simulink model "integration_MPC_model_7"  (R2023a)
settings: Solver=VariableStepAuto  StartTime=0.0  StopTime=30  FixedStep=SampleTime  RelTol=1e-3
PreLoadFcn:
  | %
  | 
  | %   Copyright 2020-2022 The MathWorks, Inc.
  | 
  | %Based on the quadcopter model used in jMAVSim
  | 
  | Ixx = 0.005; %Kgm^2
  | Iyy = 0.005;
  | Izz = 0.009;
  | 
  | 
  | inertia = diag([Ixx, Iyy, Izz]);
  | 
  | mass = 0.8; %Kg
  | g = 9.81; %m/s^2
  | 
  | armLength = 0.33/2; % length of Arm measured from center in m
  | 
  | rotorThrustMax = 4; %N
  | 
  | rotorTorqueMax = 0.05 ;%Nm
  | 
  | rotorTimeConst = 0.005 ;% time constant of rotor (motor + propeller)
  | 
  | %rotorOffset = [0 0 0]; % Rotors position offsets from Gravity center
  | 
  | dragCoeffMov = 0.01; %drag coefficient for linear motion of quadcopter
  | windVel = [0 0 0]';
  | 
  | % Initial states
  | init.posNED = [0, 0, 0]; % m
  | init.vb = [0 0 0]'; %m/s
  | init.euler = [0, 0, 0]'; %Roll Pitch Yaw Rads
  | init.angRates = [0, 0, 0]; %rad/s
  | 
  | 
  | %Computed from above values
  | rotorPositions = zeros(3,4);
  | axisD = armLength/sqrt(2);
  | rotorPositions(:,1) = [axisD, axisD, 0]';
  | rotorPositions(:,2) = [-axisD, -axisD, 0]';
  | rotorPositions(:,3) = [+axisD, -axisD, 0]';
  | rotorPositions(:,4) = [-axisD, axisD, 0]';
  | rotorDir = [-1, -1, 1, 1]; %rotation direction. +ve = clockwise
  | 
  | % Sample Time
  | SampleTime = 0.008;
  | 
  | %Gain to convert m to mm
  | m_to_mm = 1000;
  | 
  | %Gain to convert m/s^2 to mG
  | ms2_to_mg = (1/9.80665)*1000;
  | 
  | %Gain to convert m/s to cm/s
  | ms_to_cms = 100;
  | 
  | %Reference height for 'Flat Earth to LLA'
  | ref_height = -71.3232;
  | 
  | ... (+137 lines)
values from neighbouring files (symbols this model uses):
  a = 6    [integration_parameters.m]    (also in simulation_parameters.m)
  delay_tilt = 0.004    [integration_parameters.m]    (also in simulation_parameters.m)
  J = diag([0.018 0.035 0.051])    [integration_parameters.m]    (also in simulation_parameters.m)
  kf = 65    [integration_parameters.m]    (also in simulation_parameters.m)
  Lh = 0.2    [CoG_shift.m]    (also in integration_parameters.m; simulation_parameters.m)
  Lv = 0.2    [integration_parameters.m]    (also in simulation_parameters.m)
  m = 1.12    [integration_parameters.m]    (also in optimal_controller_pitching.m; simulation_parameters.m)
  N = 150    [MPC_controller_full.m]
  p_D = 0    [controller_parameters.m]    (also in integration_parameters.m)
  p_I = 0    [controller_parameters.m]    (also in integration_parameters.m)
  p_P = 0.35    [controller_parameters.m]    (also in integration_parameters.m)
  pitch_D = 0    [controller_parameters.m]    (also in integration_parameters.m)
  pitch_I = 0.05    [controller_parameters.m]    (also in integration_parameters.m = 0)
  pitch_P = 2    [controller_parameters.m]    (also in integration_parameters.m = 10)
  reference = [1 1 1 0 30 60]'    [integration_parameters.m]    (also in simulation_parameters.m = [1 1 1 0 30 40]')
  roll_D = 1    [controller_parameters.m]    (also in integration_parameters.m)
  roll_I = 0    [controller_parameters.m]    (also in integration_parameters.m)
  roll_P = 8    [controller_parameters.m]    (also in integration_parameters.m)
  s_r = [1 1 1 1 1 1]    [integration_parameters.m]    (also in simulation_parameters.m)
  Tmax = 5.5    [integration_parameters.m]    (also in simulation_parameters.m)
  toll = 1e-12    [integration_parameters.m]    (also in simulation_parameters.m)
  vy_D = 0    [controller_parameters.m]    (also in integration_parameters.m)
  vy_I = 0    [controller_parameters.m]    (also in integration_parameters.m)
  vy_P = 12    [controller_parameters.m]    (also in integration_parameters.m)
  vz_D = 0    [controller_parameters.m]    (also in integration_parameters.m)
  vz_I = 0    [controller_parameters.m]    (also in integration_parameters.m)
  vz_P = 8    [controller_parameters.m]    (also in integration_parameters.m = 9)
  x_D = 1.5    [controller_parameters.m]    (also in integration_parameters.m = 0)
  x_I = 0    [controller_parameters.m]    (also in integration_parameters.m)
  x_P = 6    [controller_parameters.m]    (also in integration_parameters.m = 1.5)
  y_D = 0.3    [controller_parameters.m]    (also in integration_parameters.m)
  y_I = 0    [controller_parameters.m]    (also in integration_parameters.m)
  y_P = 1.5    [controller_parameters.m]    (also in integration_parameters.m)
  yaw_D = 0    [controller_parameters.m]    (also in integration_parameters.m)
  yaw_I = 0    [controller_parameters.m]    (also in integration_parameters.m)
  yaw_P = 1.5    [controller_parameters.m]    (also in integration_parameters.m)
  z_D = 0    [controller_parameters.m]    (also in integration_parameters.m)
  z_I = 0    [controller_parameters.m]    (also in integration_parameters.m)
  z_P = 3    [controller_parameters.m]    (also in integration_parameters.m = 2.5)
undefined symbols (not defined in the file or in its folder): X, Y, Z
libraries: sm_lib x49, nesl_utility x29, slpidlib x9, simulink x5, simulink_extras x3, SignalEditorBlockLib x1, mpclib x1, eeGeneralControl x1
(part 3 of 4)

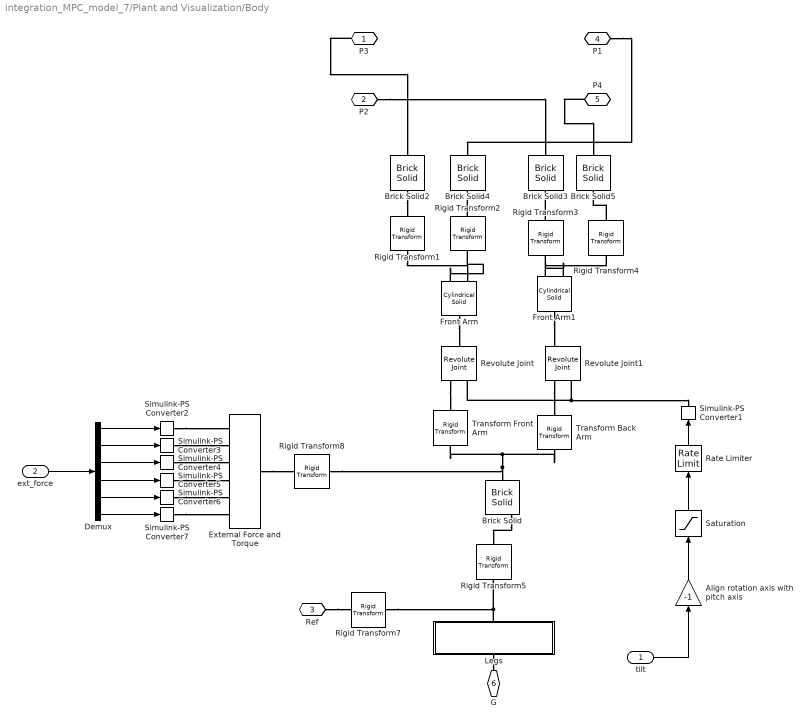
== system integration_MPC_model_7/Plant and Visualization/Body ==
  tilt : Inport
  ext_force : Inport  Port=2
  Align rotation axis with pitch axis : Gain  Gain=-1
  Brick Solid : sm_lib/Body Elements/Brick Solid  GraphicAmbientColor=[0.15 0.15 0.15 1.0]  BasedOnType=Mass  BrickDimensions=[0.1 0.5 0.05]  BrickDimensionsUnits=m  CenterOfMass=[0 0 0]  CenterOfMassUnits=m  GraphicDiffuseColor=[0.5 0.5 0.5]  Density=50  DensityUnits=kg/m^3  DoExposeReferenceFrame=on  GraphicEmissiveColor=[0.0 0.0 0.0 1.0]  ExportEntireGeometry=off  SerializedFrames=<Frames><Frame><Id>Frame2</Id><Value><Name>top</Name><Origin><Source>GeometricFeature</Source><FeatureName>+z surface</FeatureName></Origin><PrimaryAxis><DefinedDirection>+Z</DefinedDirection><Source>ReferenceFrame</Source><SourceDirection>+Z</SourceDirection><FeatureName></FeatureName></PrimaryAxis><SecondaryAxis><DefinedDirection>+X</DefinedDirection><Source>ReferenceFrame</Source><SourceDirection>+Y</SourceDirection><FeatureName></FeatureName></SecondaryAxis></Value></Frame><Frame><Id>Frame3</Id><Value><Name>bottom</Name><Origin><Source>GeometricFeature</Source><FeatureName>-z surface</FeatureName></Origin><PrimaryAxis><DefinedDirection>+Z</DefinedDirection><Source>ReferenceFrame</Source><SourceDirection>+Z</SourceDirection><FeatureName></FeatureName></PrimaryAxis><SecondaryAxis><DefinedDirection>+X</DefinedDirection><Source>ReferenceFrame</Source><SourceDirection>+X</SourceDirection><FeatureName></FeatureName></SecondaryAxis></Value></Frame></Frames>  MarkerShape=Sphere  MarkerSize=10  GraphicType=FromGeometry  InertiaType=CalculateFromGeometry  Mass=0.5  MassUnits=kg  MomentsOfInertia=[1 1 1]  MomentsOfInertiaUnits=kg*m^2  GraphicOpacity=1.0  ProductsOfInertia=[0 0 0]  ProductsOfInertiaUnits=kg*m^2  GraphicShininess=75  GraphicSpecularColor=[0.5 0.5 0.5 1.0]  GraphicVisPropType=AdvancedVisualProperties
  Brick Solid2 : sm_lib/Body Elements/Brick Solid  GraphicAmbientColor=[0.15 0.15 0.15 1.0]  BasedOnType=Mass  BrickDimensions=[0.04 0.04 0.04]  BrickDimensionsUnits=m  CenterOfMass=[0 0 0]  CenterOfMassUnits=m  GraphicDiffuseColor=[1.0 0.6 0.6]  Density=0.00001  DensityUnits=kg/m^3  DoExposeReferenceFrame=on  GraphicEmissiveColor=[0.0 0.0 0.0 1.0]  ExportEntireGeometry=off  SerializedFrames=<Frames><Frame><Id>Frame1</Id><Value><Name>top</Name><Origin><Source>GeometricFeature</Source><FeatureName>+z surface</FeatureName></Origin><PrimaryAxis><DefinedDirection>+Z</DefinedDirection><Source>ReferenceFrame</Source><SourceDirection>+Z</SourceDirection><FeatureName></FeatureName></PrimaryAxis><SecondaryAxis><DefinedDirection>+X</DefinedDirection><Source>ReferenceFrame</Source><SourceDirection>+X</SourceDirection><FeatureName></FeatureName></SecondaryAxis></Value></Frame></Frames>  MarkerShape=Sphere  MarkerSize=10  GraphicType=FromGeometry  InertiaType=CalculateFromGeometry  Mass=0.08  MassUnits=kg  MomentsOfInertia=[1 1 1]  MomentsOfInertiaUnits=kg*m^2  GraphicOpacity=1.0  ProductsOfInertia=[0 0 0]  ProductsOfInertiaUnits=kg*m^2  GraphicShininess=75  GraphicSpecularColor=[0.5 0.5 0.5 1.0]  GraphicVisPropType=SimpleVisualProperties
  Brick Solid3 : sm_lib/Body Elements/Brick Solid  GraphicAmbientColor=[0.15 0.15 0.15 1.0]  BasedOnType=Mass  BrickDimensions=[0.04 0.04 0.04]  BrickDimensionsUnits=m  CenterOfMass=[0 0 0]  CenterOfMassUnits=m  GraphicDiffuseColor=[0.4 1.0 0.4]  Density=0.00001  DensityUnits=kg/m^3  DoExposeReferenceFrame=on  GraphicEmissiveColor=[0.0 0.0 0.0 1.0]  ExportEntireGeometry=off  SerializedFrames=<Frames><Frame><Id>Frame1</Id><Value><Name>top</Name><Origin><Source>GeometricFeature</Source><FeatureName>+z surface</FeatureName></Origin><PrimaryAxis><DefinedDirection>+Z</DefinedDirection><Source>ReferenceFrame</Source><SourceDirection>+Z</SourceDirection><FeatureName></FeatureName></PrimaryAxis><SecondaryAxis><DefinedDirection>+X</DefinedDirection><Source>ReferenceFrame</Source><SourceDirection>+X</SourceDirection><FeatureName></FeatureName></SecondaryAxis></Value></Frame></Frames>  MarkerShape=Sphere  MarkerSize=10  GraphicType=FromGeometry  InertiaType=CalculateFromGeometry  Mass=0.08  MassUnits=kg  MomentsOfInertia=[1 1 1]  MomentsOfInertiaUnits=kg*m^2  GraphicOpacity=1.0  ProductsOfInertia=[0 0 0]  ProductsOfInertiaUnits=kg*m^2  GraphicShininess=75  GraphicSpecularColor=[0.5 0.5 0.5 1.0]  GraphicVisPropType=SimpleVisualProperties
  Brick Solid4 : sm_lib/Body Elements/Brick Solid  GraphicAmbientColor=[0.15 0.15 0.15 1.0]  BasedOnType=Mass  BrickDimensions=[0.04 0.04 0.04]  BrickDimensionsUnits=m  CenterOfMass=[0 0 0]  CenterOfMassUnits=m  GraphicDiffuseColor=[0.0 0.6 1.0]  Density=0.00001  DensityUnits=kg/m^3  DoExposeReferenceFrame=on  GraphicEmissiveColor=[0.0 0.0 0.0 1.0]  ExportEntireGeometry=off  SerializedFrames=<Frames><Frame><Id>Frame1</Id><Value><Name>top</Name><Origin><Source>GeometricFeature</Source><FeatureName>+z surface</FeatureName></Origin><PrimaryAxis><DefinedDirection>+Z</DefinedDirection><Source>ReferenceFrame</Source><SourceDirection>+Z</SourceDirection><FeatureName></FeatureName></PrimaryAxis><SecondaryAxis><DefinedDirection>+X</DefinedDirection><Source>ReferenceFrame</Source><SourceDirection>+X</SourceDirection><FeatureName></FeatureName></SecondaryAxis></Value></Frame></Frames>  MarkerShape=Sphere  MarkerSize=10  GraphicType=FromGeometry  InertiaType=CalculateFromGeometry  Mass=0.08  MassUnits=kg  MomentsOfInertia=[1 1 1]  MomentsOfInertiaUnits=kg*m^2  GraphicOpacity=1.0  ProductsOfInertia=[0 0 0]  ProductsOfInertiaUnits=kg*m^2  GraphicShininess=75  GraphicSpecularColor=[0.5 0.5 0.5 1.0]  GraphicVisPropType=SimpleVisualProperties
  Brick Solid5 : sm_lib/Body Elements/Brick Solid  GraphicAmbientColor=[0.15 0.15 0.15 1.0]  BasedOnType=Mass  BrickDimensions=[0.04 0.04 0.04]  BrickDimensionsUnits=m  CenterOfMass=[0 0 0]  CenterOfMassUnits=m  GraphicDiffuseColor=[0.5 0.5 0.5]  Density=0.00001  DensityUnits=kg/m^3  DoExposeReferenceFrame=on  GraphicEmissiveColor=[0.0 0.0 0.0 1.0]  ExportEntireGeometry=off  SerializedFrames=<Frames><Frame><Id>Frame1</Id><Value><Name>top</Name><Origin><Source>GeometricFeature</Source><FeatureName>+z surface</FeatureName></Origin><PrimaryAxis><DefinedDirection>+Z</DefinedDirection><Source>ReferenceFrame</Source><SourceDirection>+Z</SourceDirection><FeatureName></FeatureName></PrimaryAxis><SecondaryAxis><DefinedDirection>+X</DefinedDirection><Source>ReferenceFrame</Source><SourceDirection>+X</SourceDirection><FeatureName></FeatureName></SecondaryAxis></Value></Frame></Frames>  MarkerShape=Sphere  MarkerSize=10  GraphicType=FromGeometry  InertiaType=CalculateFromGeometry  Mass=0.08  MassUnits=kg  MomentsOfInertia=[1 1 1]  MomentsOfInertiaUnits=kg*m^2  GraphicOpacity=1.0  ProductsOfInertia=[0 0 0]  ProductsOfInertiaUnits=kg*m^2  GraphicShininess=75  GraphicSpecularColor=[0.5 0.5 0.5 1.0]  GraphicVisPropType=SimpleVisualProperties
  Demux : Demux  Outputs=6
  External Force and Torque : sm_lib/Forces and Torques/External Force and Torque  ForceResolutionFrame=AttachedFrame  EnableForceX=on  EnableForceY=on  EnableForceZ=on  EnableForce=off  TorqueResolutionFrame=AttachedFrame  EnableTorqueX=on  EnableTorqueY=on  EnableTorqueZ=on  EnableTorque=off
  Front Arm : sm_lib/Body Elements/Cylindrical Solid  GraphicAmbientColor=[0.15 0.15 0.15 1.0]  BasedOnType=Mass  CenterOfMass=[0 0 0]  CenterOfMassUnits=m  GraphicDiffuseColor=[1.0 0.0 0.2]  CylinderLength=0.4  CylinderLengthUnits=m  CylinderRadius=0.016  CylinderRadiusUnits=m  Density=0.0003  DensityUnits=g/cm^3  DoExposeReferenceFrame=on  GraphicEmissiveColor=[0.0 0.0 0.0 1.0]  ExportEntireGeometry=off  SerializedFrames=<Frames><Frame><Id>Frame1</Id><Value><Name>right</Name><Origin><Source>GeometricFeature</Source><FeatureName>top curve</FeatureName></Origin><PrimaryAxis><DefinedDirection>+Z</DefinedDirection><Source>ReferenceFrame</Source><SourceDirection>+Z</SourceDirection><FeatureName></FeatureName></PrimaryAxis><SecondaryAxis><DefinedDirection>+X</DefinedDirection><Source>ReferenceFrame</Source><SourceDirection>+X</SourceDirection><FeatureName></FeatureName></SecondaryAxis></Value></Frame><Frame><Id>Frame2</Id><Value><Name>left</Name><Origin><Source>GeometricFeature</Source><FeatureName>bottom curve</FeatureName></Origin><PrimaryAxis><DefinedDirection>+Z</DefinedDirection><Source>ReferenceFrame</Source><SourceDirection>+Z</SourceDirection><FeatureName></FeatureName></PrimaryAxis><SecondaryAxis><DefinedDirection>+X</DefinedDirection><Source>ReferenceFrame</Source><SourceDirection>+X</SourceDirection><FeatureName></FeatureName></SecondaryAxis></Value></Frame></Frames>  MarkerShape=Sphere  MarkerSize=10  GraphicType=FromGeometry  InertiaType=CalculateFromGeometry  Mass=0.1  MassUnits=kg  MomentsOfInertia=[1 1 1]  MomentsOfInertiaUnits=kg*m^2  GraphicOpacity=1.0  ProductsOfInertia=[0 0 0]  ProductsOfInertiaUnits=kg*m^2  GraphicShininess=75  GraphicSpecularColor=[0.5 0.5 0.5 1.0]  GraphicVisPropType=SimpleVisualProperties
  Front Arm1 : sm_lib/Body Elements/Cylindrical Solid  GraphicAmbientColor=[0.15 0.15 0.15 1.0]  BasedOnType=Mass  CenterOfMass=[0 0 0]  CenterOfMassUnits=m  GraphicDiffuseColor=[1.0 0.0 0.2]  CylinderLength=0.4  CylinderLengthUnits=m  CylinderRadius=0.016  CylinderRadiusUnits=m  Density=0.0003  DensityUnits=g/cm^3  DoExposeReferenceFrame=on  GraphicEmissiveColor=[0.0 0.0 0.0 1.0]  ExportEntireGeometry=off  SerializedFrames=<Frames><Frame><Id>Frame1</Id><Value><Name>right</Name><Origin><Source>GeometricFeature</Source><FeatureName>top curve</FeatureName></Origin><PrimaryAxis><DefinedDirection>+Z</DefinedDirection><Source>ReferenceFrame</Source><SourceDirection>+Z</SourceDirection><FeatureName></FeatureName></PrimaryAxis><SecondaryAxis><DefinedDirection>+X</DefinedDirection><Source>ReferenceFrame</Source><SourceDirection>+X</SourceDirection><FeatureName></FeatureName></SecondaryAxis></Value></Frame><Frame><Id>Frame2</Id><Value><Name>left</Name><Origin><Source>GeometricFeature</Source><FeatureName>bottom curve</FeatureName></Origin><PrimaryAxis><DefinedDirection>+Z</DefinedDirection><Source>ReferenceFrame</Source><SourceDirection>+Z</SourceDirection><FeatureName></FeatureName></PrimaryAxis><SecondaryAxis><DefinedDirection>+X</DefinedDirection><Source>ReferenceFrame</Source><SourceDirection>+X</SourceDirection><FeatureName></FeatureName></SecondaryAxis></Value></Frame></Frames>  MarkerShape=Sphere  MarkerSize=10  GraphicType=FromGeometry  InertiaType=CalculateFromGeometry  Mass=0.1  MassUnits=kg  MomentsOfInertia=[1 1 1]  MomentsOfInertiaUnits=kg*m^2  GraphicOpacity=1.0  ProductsOfInertia=[0 0 0]  ProductsOfInertiaUnits=kg*m^2  GraphicShininess=75  GraphicSpecularColor=[0.5 0.5 0.5 1.0]  GraphicVisPropType=SimpleVisualProperties
  Legs : Subsystem
  Rate Limiter : RateLimiter  RisingSlewLimit=4.2  FallingSlewLimit=-4.2
  Revolute Joint : sm_lib/Joints/Revolute Joint  JointMode=Normal  SenseConstraintForce=off  SenseConstraintForceX=off  SenseConstraintForceY=off  SenseConstraintForceZ=off  SenseConstraintTorque=off  SenseConstraintTorqueX=off  SenseConstraintTorqueY=off  SenseConstraintTorqueZ=off  SenseTotalForce=off  SenseTotalForceX=off  SenseTotalForceY=off  SenseTotalForceZ=off  SenseTotalTorque=off  SenseTotalTorqueX=off  SenseTotalTorqueY=off  SenseTotalTorqueZ=off  CompositeWrenchDir=FollowerOnBase  CompositeWrenchFrame=BaseFrame  EquilibriumPosition=0  EquilibriumPositionUnits=deg  SpringStiffness=0  SpringStiffnessUnits=N*m/deg  DampingCoefficient=0  DampingCoefficientUnits=N*m/(deg/s)  TorqueActuationMode=ComputedTorque  MotionActuationMode=InputMotion  SensePosition=off  SenseVelocity=off  SenseAcceleration=off  SenseTorqueForce=off  SenseLowerLimitTorqueForce=off  SenseUpperLimitTorqueForce=off  LowerLimitSpecify=on  LowerLimitBound=-45  LowerLimitBoundUnits=deg  LowerLimitStiffness=1e4  LowerLimitStiffnessUnits=N*m/deg  LowerLimitDamping=10  LowerLimitDampingUnits=N*m/(deg/s)  LowerLimitTransitionRegionWidth=0.1  LowerLimitTransitionRegionWidthUnits=deg  UpperLimitSpecify=on  UpperLimitBound=45  UpperLimitBoundUnits=deg  UpperLimitStiffness=1e4  UpperLimitStiffnessUnits=N*m/deg  UpperLimitDamping=10  UpperLimitDampingUnits=N*m/(deg/s)  UpperLimitTransitionRegionWidth=0.1  UpperLimitTransitionRegionWidthUnits=deg  PositionTargetSpecify=off  PositionTargetPriority=High  PositionTargetValue=0  PositionTargetValueUnits=deg  VelocityTargetSpecify=off  VelocityTargetPriority=High  VelocityTargetValue=0  VelocityTargetValueUnits=deg/s
  Revolute Joint1 : sm_lib/Joints/Revolute Joint  JointMode=Normal  SenseConstraintForce=off  SenseConstraintForceX=off  SenseConstraintForceY=off  SenseConstraintForceZ=off  SenseConstraintTorque=off  SenseConstraintTorqueX=off  SenseConstraintTorqueY=off  SenseConstraintTorqueZ=off  SenseTotalForce=off  SenseTotalForceX=off  SenseTotalForceY=off  SenseTotalForceZ=off  SenseTotalTorque=off  SenseTotalTorqueX=off  SenseTotalTorqueY=off  SenseTotalTorqueZ=off  CompositeWrenchDir=FollowerOnBase  CompositeWrenchFrame=BaseFrame  EquilibriumPosition=0  EquilibriumPositionUnits=deg  SpringStiffness=0  SpringStiffnessUnits=N*m/deg  DampingCoefficient=0  DampingCoefficientUnits=N*m/(deg/s)  TorqueActuationMode=ComputedTorque  MotionActuationMode=InputMotion  SensePosition=on  SenseVelocity=off  SenseAcceleration=off  SenseTorqueForce=off  SenseLowerLimitTorqueForce=off  SenseUpperLimitTorqueForce=off  LowerLimitSpecify=on  LowerLimitBound=-45  LowerLimitBoundUnits=deg  LowerLimitStiffness=1e4  LowerLimitStiffnessUnits=N*m/deg  LowerLimitDamping=10  LowerLimitDampingUnits=N*m/(deg/s)  LowerLimitTransitionRegionWidth=0.1  LowerLimitTransitionRegionWidthUnits=deg  UpperLimitSpecify=on  UpperLimitBound=45  UpperLimitBoundUnits=deg  UpperLimitStiffness=1e4  UpperLimitStiffnessUnits=N*m/deg  UpperLimitDamping=10  UpperLimitDampingUnits=N*m/(deg/s)  UpperLimitTransitionRegionWidth=0.1  UpperLimitTransitionRegionWidthUnits=deg  PositionTargetSpecify=off  PositionTargetPriority=High  PositionTargetValue=0  PositionTargetValueUnits=deg  VelocityTargetSpecify=off  VelocityTargetPriority=High  VelocityTargetValue=0  VelocityTargetValueUnits=deg/s
  Rigid Transform1 : sm_lib/Frames and Transforms/Rigid Transform  TranslationMethod=None  TranslationStandardOffset=0  TranslationStandardOffsetUnits=m  TranslationStandardAxis=+Z  TranslationCartesianOffset=[0.2 0 0]  TranslationCartesianOffsetUnits=m  TranslationROffset=0  TranslationROffsetUnits=m  TranslationZOffset=0  TranslationZOffsetUnits=m  TranslationThetaOffset=0  TranslationThetaOffsetUnits=deg  RotationMethod=RotationSequence  RotationAngleUnits=deg  RotationStandardAxis=+X  RotationAngle=180  RotationArbitraryAxis=[0 0 1]  FollAlignAxisA=+X  BaseAlignAxisA=+Y  FollAlignAxisB=+Y  BaseAlignAxisB=+Z  RotationSequenceAxes=FollowerAxes  RotationSequence=ZYZ  RotationSequenceAngles=[90 180 0]  RotationSequenceAnglesUnits=deg  RotationMatrix=[1 0 0; 0 1 0; 0 0 1]  Quaternion=[1 0 0 0]
  Rigid Transform2 : sm_lib/Frames and Transforms/Rigid Transform  TranslationMethod=None  TranslationStandardOffset=0  TranslationStandardOffsetUnits=m  TranslationStandardAxis=+Z  TranslationCartesianOffset=[0.2 0 0]  TranslationCartesianOffsetUnits=m  TranslationROffset=0  TranslationROffsetUnits=m  TranslationZOffset=0  TranslationZOffsetUnits=m  TranslationThetaOffset=0  TranslationThetaOffsetUnits=deg  RotationMethod=StandardAxis  RotationAngleUnits=deg  RotationStandardAxis=+Z  RotationAngle=90  RotationArbitraryAxis=[0 0 1]  FollAlignAxisA=+X  BaseAlignAxisA=+Y  FollAlignAxisB=+Y  BaseAlignAxisB=+Z  RotationSequenceAxes=FollowerAxes  RotationSequence=XYX  RotationSequenceAngles=[0 0 0]  RotationSequenceAnglesUnits=deg  RotationMatrix=[1 0 0; 0 1 0; 0 0 1]  Quaternion=[1 0 0 0]
  Rigid Transform3 : sm_lib/Frames and Transforms/Rigid Transform  TranslationMethod=None  TranslationStandardOffset=0  TranslationStandardOffsetUnits=m  TranslationStandardAxis=+Z  TranslationCartesianOffset=[0.2 0 0]  TranslationCartesianOffsetUnits=m  TranslationROffset=0  TranslationROffsetUnits=m  TranslationZOffset=0  TranslationZOffsetUnits=m  TranslationThetaOffset=0  TranslationThetaOffsetUnits=deg  RotationMethod=RotationSequence  RotationAngleUnits=deg  RotationStandardAxis=+X  RotationAngle=180  RotationArbitraryAxis=[0 0 1]  FollAlignAxisA=+X  BaseAlignAxisA=+Y  FollAlignAxisB=+Y  BaseAlignAxisB=+Z  RotationSequenceAxes=FollowerAxes  RotationSequence=ZYZ  RotationSequenceAngles=[90 180 0]  RotationSequenceAnglesUnits=deg  RotationMatrix=[1 0 0; 0 1 0; 0 0 1]  Quaternion=[1 0 0 0]
  Rigid Transform4 : sm_lib/Frames and Transforms/Rigid Transform  TranslationMethod=None  TranslationStandardOffset=0  TranslationStandardOffsetUnits=m  TranslationStandardAxis=+Z  TranslationCartesianOffset=[0.2 0 0]  TranslationCartesianOffsetUnits=m  TranslationROffset=0  TranslationROffsetUnits=m  TranslationZOffset=0  TranslationZOffsetUnits=m  TranslationThetaOffset=0  TranslationThetaOffsetUnits=deg  RotationMethod=StandardAxis  RotationAngleUnits=deg  RotationStandardAxis=+Z  RotationAngle=90  RotationArbitraryAxis=[0 0 1]  FollAlignAxisA=+X  BaseAlignAxisA=+Y  FollAlignAxisB=+Y  BaseAlignAxisB=+Z  RotationSequenceAxes=FollowerAxes  RotationSequence=XYX  RotationSequenceAngles=[0 0 0]  RotationSequenceAnglesUnits=deg  RotationMatrix=[1 0 0; 0 1 0; 0 0 1]  Quaternion=[1 0 0 0]
  Rigid Transform5 : sm_lib/Frames and Transforms/Rigid Transform  TranslationMethod=None  TranslationStandardOffset=0  TranslationStandardOffsetUnits=m  TranslationStandardAxis=+Z  TranslationCartesianOffset=[0 0 0]  TranslationCartesianOffsetUnits=m  TranslationROffset=0  TranslationROffsetUnits=m  TranslationZOffset=0  TranslationZOffsetUnits=m  TranslationThetaOffset=0  TranslationThetaOffsetUnits=deg  RotationMethod=RotationSequence  RotationAngleUnits=deg  RotationStandardAxis=-Z  RotationAngle=90  RotationArbitraryAxis=[0 0 1]  FollAlignAxisA=+X  BaseAlignAxisA=+Y  FollAlignAxisB=+Y  BaseAlignAxisB=+Z  RotationSequenceAxes=FollowerAxes  RotationSequence=ZYX  RotationSequenceAngles=[-90 180 0]  RotationSequenceAnglesUnits=deg  RotationMatrix=[1 0 0; 0 1 0; 0 0 1]  Quaternion=[1 0 0 0]
  Rigid Transform7 : sm_lib/Frames and Transforms/Rigid Transform  TranslationMethod=None  TranslationStandardOffset=0  TranslationStandardOffsetUnits=m  TranslationStandardAxis=+Z  TranslationCartesianOffset=[0 0 0]  TranslationCartesianOffsetUnits=m  TranslationROffset=0  TranslationROffsetUnits=m  TranslationZOffset=0  TranslationZOffsetUnits=m  TranslationThetaOffset=0  TranslationThetaOffsetUnits=deg  RotationMethod=StandardAxis  RotationAngleUnits=deg  RotationStandardAxis=+X  RotationAngle=180  RotationArbitraryAxis=[0 0 1]  FollAlignAxisA=+X  BaseAlignAxisA=+Y  FollAlignAxisB=+Y  BaseAlignAxisB=+Z  RotationSequenceAxes=FollowerAxes  RotationSequence=XYX  RotationSequenceAngles=[0 0 0]  RotationSequenceAnglesUnits=deg  RotationMatrix=[1 0 0; 0 1 0; 0 0 1]  Quaternion=[1 0 0 0]
  Rigid Transform8 : sm_lib/Frames and Transforms/Rigid Transform  TranslationMethod=None  TranslationStandardOffset=0  TranslationStandardOffsetUnits=m  TranslationStandardAxis=+Z  TranslationCartesianOffset=[0 0 0]  TranslationCartesianOffsetUnits=m  TranslationROffset=0  TranslationROffsetUnits=m  TranslationZOffset=0  TranslationZOffsetUnits=m  TranslationThetaOffset=0  TranslationThetaOffsetUnits=deg  RotationMethod=StandardAxis  RotationAngleUnits=deg  RotationStandardAxis=+Z  RotationAngle=90  RotationArbitraryAxis=[0 0 1]  FollAlignAxisA=+X  BaseAlignAxisA=+Y  FollAlignAxisB=+Y  BaseAlignAxisB=+Z  RotationSequenceAxes=FollowerAxes  RotationSequence=XYX  RotationSequenceAngles=[0 0 0]  RotationSequenceAnglesUnits=deg  RotationMatrix=[1 0 0; 0 1 0; 0 0 1]  Quaternion=[1 0 0 0]
  Saturation : Saturate  UpperLimit=1.6  LowerLimit=-1.6
  Simulink-PS Converter{1..7} (7 alike) : nesl_utility/Simulink-PS Converter  PhysicalDomain=network_engine_domain  SubClassName=ps_input  LeftPortType=input  RightPortType=output  PseudoPeriodic=off  Frequencies=[]  NoiseDistribution=none  NoiseParameters=[]  Unit=1  AffineConversion=off  FilteringAndDerivatives=filter  SimscapeFilterOrder=2  InputFilterTimeConstant=0.001  UdotUserProvided=0
  Transform Back Arm : sm_lib/Frames and Transforms/Rigid Transform  TranslationMethod=Cartesian  TranslationStandardOffset=0  TranslationStandardOffsetUnits=m  TranslationStandardAxis=+Z  TranslationCartesianOffset=[0 -0.2 0]  TranslationCartesianOffsetUnits=m  TranslationROffset=0  TranslationROffsetUnits=m  TranslationZOffset=0  TranslationZOffsetUnits=m  TranslationThetaOffset=0  TranslationThetaOffsetUnits=deg  RotationMethod=StandardAxis  RotationAngleUnits=deg  RotationStandardAxis=+Y  RotationAngle=90  RotationArbitraryAxis=[0 0 1]  FollAlignAxisA=+X  BaseAlignAxisA=+Y  FollAlignAxisB=+Y  BaseAlignAxisB=+Z  RotationSequenceAxes=FollowerAxes  RotationSequence=XYX  RotationSequenceAngles=[90 180 0]  RotationSequenceAnglesUnits=deg  RotationMatrix=[1 0 0; 0 1 0; 0 0 1]  Quaternion=[1 0 0 0]
  Transform Front Arm : sm_lib/Frames and Transforms/Rigid Transform  TranslationMethod=Cartesian  TranslationStandardOffset=0  TranslationStandardOffsetUnits=m  TranslationStandardAxis=+Z  TranslationCartesianOffset=[0 0.2 0]  TranslationCartesianOffsetUnits=m  TranslationROffset=0  TranslationROffsetUnits=m  TranslationZOffset=0  TranslationZOffsetUnits=m  TranslationThetaOffset=0  TranslationThetaOffsetUnits=deg  RotationMethod=StandardAxis  RotationAngleUnits=deg  RotationStandardAxis=+Y  RotationAngle=90  RotationArbitraryAxis=[0 0 1]  FollAlignAxisA=+X  BaseAlignAxisA=+Y  FollAlignAxisB=+Y  BaseAlignAxisB=+Z  RotationSequenceAxes=FollowerAxes  RotationSequence=XYX  RotationSequenceAngles=[90 180 0]  RotationSequenceAnglesUnits=deg  RotationMatrix=[1 0 0; 0 1 0; 0 0 1]  Quaternion=[1 0 0 0]
  "P3 " : PMIOPort  Side=Left
  P2 : PMIOPort  Port=2  Side=Left
  Ref : PMIOPort  Port=3  Side=Left
  P1 : PMIOPort  Port=4  Side=Right
  P4 : PMIOPort  Port=5  Side=Right
  G : PMIOPort  Port=6  Side=Right
  wires:
  Saturation/1 -> Rate Limiter/1
  Rate Limiter/1 -> Simulink-PS Converter1/1
  Align rotation axis with pitch axis/1 -> Saturation/1
  tilt/1 -> Align rotation axis with pitch axis/1
  Demux/2 -> Simulink-PS Converter3/1
  Demux/6 -> Simulink-PS Converter7/1
  Demux/5 -> Simulink-PS Converter6/1
  Demux/3 -> Simulink-PS Converter4/1
  Demux/4 -> Simulink-PS Converter5/1
  ext_force/1 -> Demux/1
  Demux/1 -> Simulink-PS Converter2/1
  connections:
  Transform Front Arm/LConn1 -- Rigid Transform8/LConn1 -- Brick Solid/RConn1 -- Transform Back Arm/LConn1
  Revolute Joint/LConn2 -- Revolute Joint1/LConn2 -- Simulink-PS Converter1/RConn1
  Legs/LConn1 -- Rigid Transform7/RConn1 -- Rigid Transform5/LConn1
  Rigid Transform1/LConn1 -- Front Arm/LConn2
  Rigid Transform4/RConn1 -- Brick Solid5/RConn1
  Rigid Transform3/RConn1 -- Brick Solid3/RConn1
  Front Arm/RConn1 -- Revolute Joint/RConn1
  Front Arm1/RConn1 -- Revolute Joint1/RConn1
  Brick Solid/LConn2 -- Rigid Transform5/RConn1
  Rigid Transform2/RConn1 -- Brick Solid4/RConn1
  Front Arm/LConn1 -- Rigid Transform2/LConn1
  Revolute Joint1/LConn1 -- Transform Back Arm/RConn1
  Revolute Joint/LConn1 -- Transform Front Arm/RConn1
  Brick Solid2/RConn1 -- Rigid Transform1/RConn1
  Front Arm1/LConn1 -- Rigid Transform4/LConn1
  Front Arm1/LConn2 -- Rigid Transform3/LConn1
  Legs/RConn1 -- G/RConn1
  "P3 "/RConn1 -- Brick Solid2/LConn1
  P1/RConn1 -- Brick Solid4/LConn1
  P2/RConn1 -- Brick Solid3/LConn1
  P4/RConn1 -- Brick Solid5/LConn1
  Ref/RConn1 -- Rigid Transform7/LConn1
  Simulink-PS Converter3/RConn1 -- External Force and Torque/LConn2
  Simulink-PS Converter2/RConn1 -- External Force and Torque/LConn1
  Simulink-PS Converter7/RConn1 -- External Force and Torque/LConn6
  Simulink-PS Converter5/RConn1 -- External Force and Torque/LConn4
  Simulink-PS Converter6/RConn1 -- External Force and Torque/LConn5
  Simulink-PS Converter4/RConn1 -- External Force and Torque/LConn3
  External Force and Torque/RConn1 -- Rigid Transform8/RConn1

== system integration_MPC_model_7/Plant and Visualization/Create States Bus ==
  Ve : Inport
  Xe : Inport  Port=2
  pqr : Inport  Port=3
  rpy : Inport  Port=4
  acc_lnav : Inport  Port=5
  Bus Creator : BusCreator  Inputs=15
  Demux{,1..4} (5 alike) : Demux  Outputs=3
  Matrix Multiply4 : Product  Multiplication=Matrix(*)
  Mux1 : Mux  Inputs=2
  "Rotation mat " : MATLAB Function  TreatAsAtomicUnit=on
  Scope : Scope
  Selector : Selector  InputPortWidth=3  IndexOptions=Index vector (dialog)  Indices=[1 2]  OutputSizes=1
  Selector1 : Selector  InputPortWidth=3  IndexOptions=Index vector (dialog)  Indices=[3]  OutputSizes=1
  To Workspace : ToWorkspace  VariableName=actual  SaveFormat=Timeseries  SampleTime=-1
  States : Outport
  wires:
  Demux1/1 -> Bus Creator/1  "X"
  Demux1/2 -> Bus Creator/2  "Y"
  rpy/1 -> Demux2/1
  Demux2/2 -> Bus Creator/5  "pitch"
  Demux3/2 -> Bus Creator/8  "dy"
  Demux2/3 -> "Rotation mat "/1(psi), Bus Creator/6  "yaw"
  pqr/1 -> Demux4/1
  Ve/1 -> Demux3/1
  Demux2/1 -> Bus Creator/4  "roll"
  Demux1/3 -> Bus Creator/3  "Z"
  Demux3/1 -> Bus Creator/7  "dx"
  Demux4/2 -> Scope/1, Bus Creator/11  "q"
  Demux3/3 -> Bus Creator/9  "dz"
  Demux4/3 -> Bus Creator/12  "r"
  Demux4/1 -> Bus Creator/10  "p"
  Bus Creator/1 -> To Workspace/1, States/1
  Xe/1 -> Selector/1, Selector1/1
  acc_lnav/1 -> Demux/1
  Demux/3 -> Bus Creator/15  "ddz"
  Demux/2 -> Bus Creator/14  "ddy"
  Demux/1 -> Bus Creator/13  "ddx"
  Selector1/1 -> Mux1/2
  Matrix Multiply4/1 -> Mux1/1
  Selector/1 -> Matrix Multiply4/2
  "Rotation mat "/1(R) -> Matrix Multiply4/1
  Mux1/1 -> Demux1/1

== system integration_MPC_model_7/Plant and Visualization/Ground ==
  Ground : Subsystem  mask{waypoints=waypoints}
      mask prompts: waypoints "Waypoints [xyz] (m)"
      mask init:
      | plane_x = max(waypoints(1,:))-min(waypoints(1,:))+6;
      | plane_y = max(waypoints(2,:))-min(waypoints(2,:))+6;
      | 
      | offset_x = plane_x/2+min(waypoints(1,:))-3;
      | offset_y = plane_y/2+min(waypoints(2,:))-3;
  Infinite Plane : sm_lib/Curves and Surfaces/Infinite Plane  GraphicType=None  GraphicPlaneWidth=1  GraphicPlaneWidthUnits=m  GraphicPlaneHeight=1  GraphicPlaneHeightUnits=m  GraphicVisPropType=SimpleVisualProperties  GraphicDiffuseColor=[0.5 0.5 0.5]  GraphicOpacity=0  GraphicSpecularColor=[0.5 0.5 0.5 1.0]  GraphicAmbientColor=[0.15 0.15 0.15 1.0]  GraphicEmissiveColor=[0.0 0.0 0.0 1.0]  GraphicShininess=75
  W : PMIOPort  Side=Right
  G : PMIOPort  Port=2  Side=Left
  connections:
  W/RConn1 -- Ground/LConn1
  Infinite Plane/LConn1 -- Ground/RConn1
  Infinite Plane/RConn1 -- G/RConn1

== system integration_MPC_model_7/Plant and Visualization/Motor allocation ==
  actuators : Inport
  Bus Creator{,1..3} (4 alike) : BusCreator  Inputs=2
  Demux1 : Demux
  Demux5 : Demux
  Gain : Gain  Gain=1/kf
  Gain1 : Gain  Gain=-1
  Gain2 : Gain  Gain=-1
  M1 : Outport
  M2 : Outport  Port=2
  M3 : Outport  Port=3
  M4 : Outport  Port=4
  wires:
  Demux1/2 -> Bus Creator2/1
  actuators/1 -> Gain/1, Demux1/1
  Gain1/1 -> Bus Creator1/2
  Demux1/4 -> Bus Creator3/1
  Gain/1 -> Demux5/1
  Demux1/3 -> Bus Creator1/1
  Demux5/3 -> Gain1/1
  Demux5/2 -> Bus Creator2/2
  Demux5/1 -> Gain2/1
  Demux5/4 -> Bus Creator3/2
  Gain2/1 -> Bus Creator/2
  Demux1/1 -> Bus Creator/1
  Bus Creator/1 -> M1/1
  Bus Creator3/1 -> M4/1
  Bus Creator2/1 -> M3/1
  Bus Creator1/1 -> M2/1

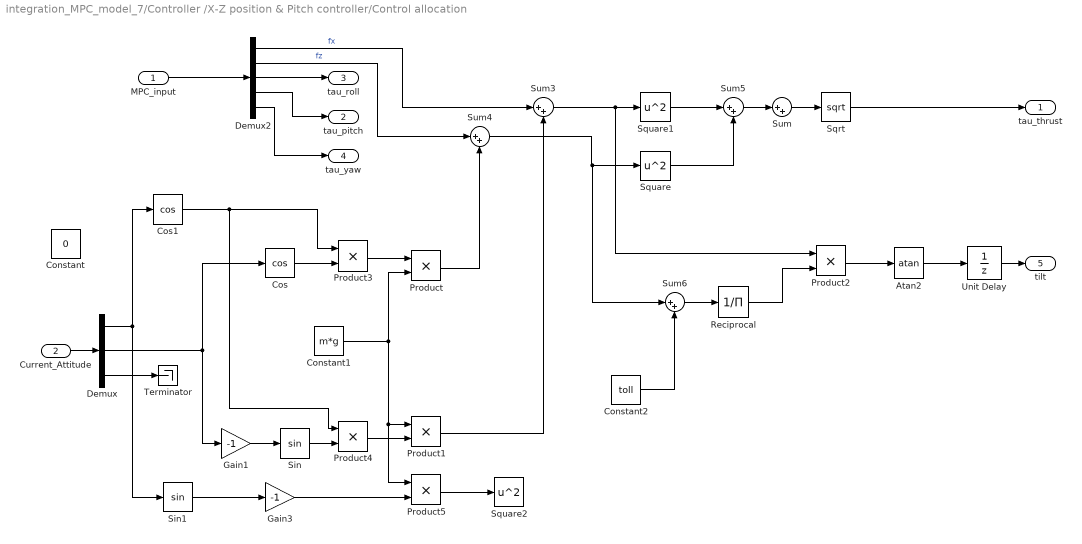
== system integration_MPC_model_7/Controller /X-Z position & Pitch controller/Control allocation ==
  MPC_input : Inport
  Current_Attitude : Inport  Port=2
  Atan2 : Trigonometry  Operator=atan
  Constant : Constant  Value=0
  Constant1 : Constant  Value=m*g
  Constant2 : Constant  Value=toll
  Cos : Trigonometry  Operator=cos
  Cos1 : Trigonometry  Operator=cos
  Demux : Demux  Outputs=3
  Demux2 : Demux  Outputs=5
  Gain1 : Gain  Gain=-1
  Gain3 : Gain  Gain=-1
  Product{,1..5} (6 alike) : Product
  Reciprocal : Product  Inputs=/
  Sin : Trigonometry
  Sin1 : Trigonometry
  Sqrt : Sqrt
  Square : Math  Operator=square
  Square1 : Math  Operator=square
  Square2 : Math  Operator=square
  Sum{,3..6} (5 alike) : Sum  Inputs=|++
  Terminator : Terminator
  Unit Delay : UnitDelay  SampleTime=delay_tilt  HasFrameUpgradeWarning=on
  tau_thrust : Outport
  tau_pitch : Outport  Port=2
  tau_roll : Outport  Port=3
  tau_yaw : Outport  Port=4
  tilt : Outport  Port=5
  wires:
  Square1/1 -> Sum5/1
  Atan2/1 -> Unit Delay/1
  Product1/1 -> Sum3/2
  Sum6/1 -> Reciprocal/1
  Sqrt/1 -> tau_thrust/1
  Product/1 -> Sum4/2
  Square/1 -> Sum5/2
  Sum3/1 -> Product2/1, Square1/1
  Constant2/1 -> Sum6/2
  Demux2/1 -> Sum3/1  "fx"
  Demux2/2 -> Sum4/1  "fz"
  Gain1/1 -> Sin/1
  Constant1/1 -> Product/2, Product5/1, Product1/1
  Reciprocal/1 -> Product2/2
  Sum4/1 -> Sum6/1, Square/1
  MPC_input/1 -> Demux2/1
  Product2/1 -> Atan2/1
  Unit Delay/1 -> tilt/1
  Demux2/4 -> tau_pitch/1
  Demux2/5 -> tau_yaw/1
  Demux2/3 -> tau_roll/1
  Current_Attitude/1 -> Demux/1
  Demux/3 -> Terminator/1
  Product3/1 -> Product/1
  Cos/1 -> Product3/2
  Cos1/1 -> Product4/1, Product3/1
  Product4/1 -> Product1/2
  Sin/1 -> Product4/2
  Sin1/1 -> Gain3/1
  Product5/1 -> Square2/1
  Sum5/1 -> Sum/1
  Sum/1 -> Sqrt/1
  Gain3/1 -> Product5/2
  Demux/2 -> Gain1/1, Cos/1
  Demux/1 -> Cos1/1, Sin1/1

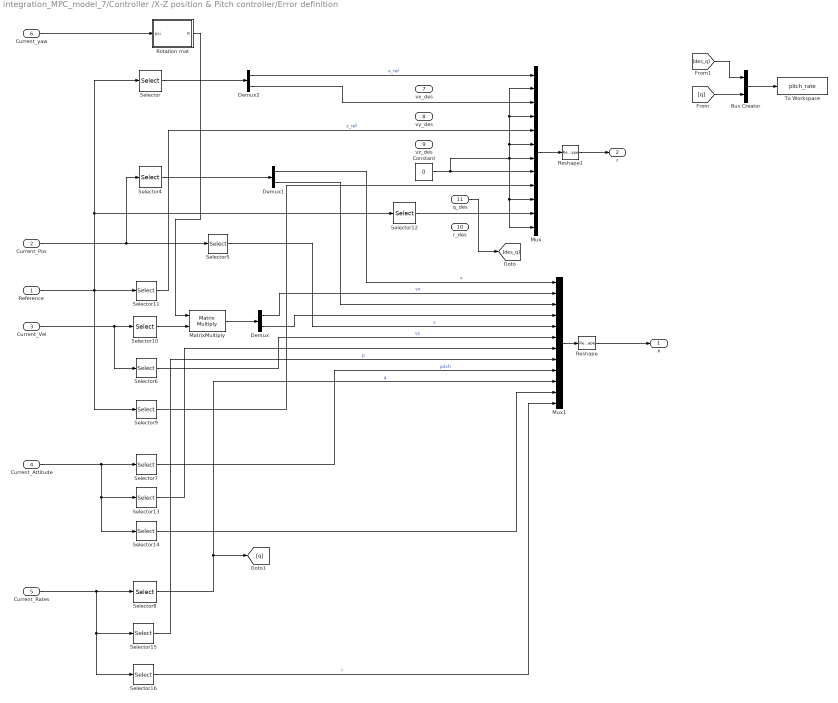
== system integration_MPC_model_7/Controller /X-Z position & Pitch controller/Error definition ==
  Reference : Inport
  Current_Pos : Inport  Port=2
  Current_Vel : Inport  Port=3
  Current_Attitude : Inport  Port=4
  Current_Rates : Inport  Port=5
  Current_yaw : Inport  Port=6
  vx_des : Inport  Port=7
  vy_des : Inport  Port=8
  vz_des : Inport  Port=9
  r_des : Inport  Port=10
  q_des : Inport  Port=11
  Bus Creator : BusCreator  Inputs=2
  Constant : Constant  Value=0
  Demux : Demux  Outputs=2
  Demux1 : Demux  Outputs=2
  Demux2 : Demux  Outputs=2
  MatrixMultiply : Product  Multiplication=Matrix(*)
  Mux : Mux  Inputs=12
  Mux1 : Mux  Inputs=12
  Reshape : Reshape  OutputDimensionality=Column vector (2-D)
  Reshape1 : Reshape  OutputDimensionality=Column vector (2-D)
  "Rotation mat " : MATLAB Function  TreatAsAtomicUnit=on
  Selector : Selector  InputPortWidth=6  IndexOptions=Index vector (dialog)  Indices=[1 2]  OutputSizes=1
  Selector10 : Selector  InputPortWidth=3  IndexOptions=Index vector (dialog)  Indices=[1 2]  OutputSizes=1
  Selector11 : Selector  InputPortWidth=6  IndexOptions=Index vector (dialog)  Indices=[3]  OutputSizes=1
  Selector12 : Selector  InputPortWidth=6  IndexOptions=Index vector (dialog)  Indices=[6]  OutputSizes=1
  Selector13 : Selector  InputPortWidth=3  IndexOptions=Index vector (dialog)  Indices=[1]  OutputSizes=1
  Selector{5..6,14,16} (4 alike) : Selector  InputPortWidth=3  IndexOptions=Index vector (dialog)  Indices=[3]  OutputSizes=1
  Selector15 : Selector  InputPortWidth=3  IndexOptions=Index vector (dialog)  Indices=[1]  OutputSizes=1
  Selector4 : Selector  InputPortWidth=3  IndexOptions=Index vector (dialog)  Indices=[1 2]  OutputSizes=1
  Selector7 : Selector  InputPortWidth=3  IndexOptions=Index vector (dialog)  Indices=[2]  OutputSizes=1
  Selector8 : Selector  InputPortWidth=3  IndexOptions=Index vector (dialog)  Indices=[2]  OutputSizes=1
  Selector9 : Selector  InputPortWidth=6  IndexOptions=Index vector (dialog)  Indices=[5]  OutputSizes=1
  To Workspace : ToWorkspace  VariableName=pitch_rate  SaveFormat=Timeseries  SampleTime=-1
  x : Outport
  r : Outport  Port=2
  wires:
  Current_Rates/1 -> Selector16/1, Selector15/1, Selector8/1
  Current_Attitude/1 -> Selector13/1, Selector14/1, Selector7/1
  Selector9/1 -> Mux/9
  Reference/1 -> Selector/1, Selector12/1, Selector11/1, Selector9/1
  Current_Vel/1 -> Selector10/1, Selector6/1
  Selector7/1 -> Mux1/9  "pitch"
  Selector/1 -> Demux2/1
  Current_Pos/1 -> Selector5/1, Selector4/1
  Selector8/1 -> [q], Mux1/10  "q"
  Mux/1 -> Reshape1/1
  Mux1/1 -> Reshape/1
  Reshape/1 -> x/1
  Reshape1/1 -> r/1
  Selector4/1 -> Demux1/1
  Current_yaw/1 -> "Rotation mat "/1(psi)
  Selector10/1 -> MatrixMultiply/2
  MatrixMultiply/1 -> Demux/1
  "Rotation mat "/1(R) -> MatrixMultiply/1
  Bus Creator/1 -> To Workspace/1
  [des_q] -> Bus Creator/1
  [q] -> Bus Creator/2
  Demux2/1 -> Mux/1  "x_ref"
  Demux1/1 -> Mux1/1  "x"
  Selector5/1 -> Mux1/5  "z"
  Constant/1 -> Mux/8, Mux/4, Mux/2, Mux/6, Mux/10, Mux/12, Mux/7
  Selector11/1 -> Mux/5  "z_ref"
  Selector12/1 -> Mux/11
  Selector6/1 -> Mux1/6  "vz"
  Demux/1 -> Mux1/2  "vx"
  Selector13/1 -> Mux1/7
  Selector14/1 -> Mux1/11
  Selector15/1 -> Mux1/8  "p"
  Selector16/1 -> Mux1/12  "r"
  Demux/2 -> Mux1/4
  Demux1/2 -> Mux1/3
  Demux2/2 -> Mux/3
  q_des/1 -> [des_q]

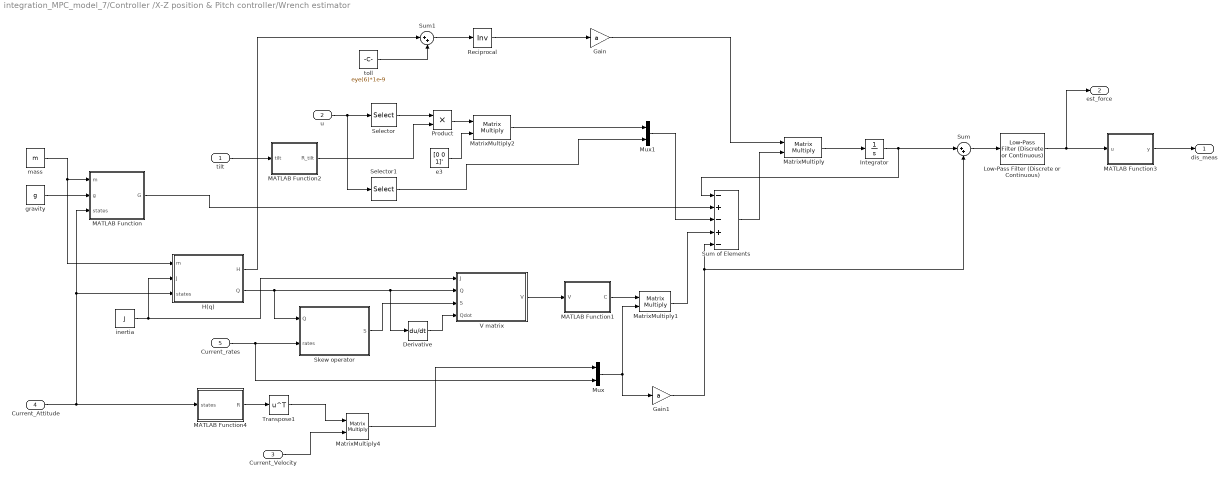
== system integration_MPC_model_7/Controller /X-Z position & Pitch controller/Wrench estimator ==
  tilt : Inport
  u : Inport  Port=2
  Current_Velocity : Inport  Port=3
  Current_Attitude : Inport  Port=4
  Current_rates : Inport  Port=5
  Derivative : Derivative
  Gain : Gain  Gain=a
  Gain1 : Gain  Gain=a
  H(q) : MATLAB Function  TreatAsAtomicUnit=on
  Integrator : Integrator
  Low-Pass Filter (Discrete or Continuous) : eeGeneralControl/Low-Pass Filter (Discrete or Continuous)  K=1  T=1  B=inf  A=-inf  init_option=Inherited from block input  x0=0  Ts=-1
  MATLAB Function : MATLAB Function  TreatAsAtomicUnit=on
  MATLAB Function1 : MATLAB Function  TreatAsAtomicUnit=on
  MATLAB Function2 : MATLAB Function  TreatAsAtomicUnit=on
  MATLAB Function3 : MATLAB Function  TreatAsAtomicUnit=on
  MATLAB Function4 : MATLAB Function  TreatAsAtomicUnit=on
  MatrixMultiply{,1..2,4} (4 alike) : Product  Multiplication=Matrix(*)
  Mux : Mux  Inputs=2
  Mux1 : Mux  Inputs=2
  Product : Product
  Reciprocal : Product  Inputs=/  Multiplication=Matrix(*)
  Selector : Selector  InputPortWidth=4  IndexOptions=Index vector (dialog)  Indices=[1]  OutputSizes=1
  Selector1 : Selector  InputPortWidth=4  IndexOptions=Index vector (dialog)  Indices=[2:4]  OutputSizes=1
  Skew operator : MATLAB Function  TreatAsAtomicUnit=on
  Sum : Sum  Inputs=|++
  Sum of Elements : Sum  Inputs=-+-+-
  Sum1 : Sum  Inputs=|++
  Transpose1 : Math  Operator=transpose
  V matrix : MATLAB Function  TreatAsAtomicUnit=on
  e3 : Constant  Value=[0 0 1]'  VectorParams1D=off
  gravity : Constant  Value=g
  inertia : Constant  Value=J  VectorParams1D=off
  mass : Constant  Value=m  VectorParams1D=off
  toll : Constant  Value=eye(6)*1e-9
  dis_meas : Outport
  est_force : Outport  Port=2
  wires:
  toll/1 -> Sum1/2
  MATLAB Function1/1(C) -> MatrixMultiply1/1
  MatrixMultiply/1 -> Integrator/1
  Mux1/1 -> Sum of Elements/3
  MATLAB Function2/1(R_tilt) -> Product/2
  Current_rates/1 -> Mux/2, Skew operator/2(rates)
  MatrixMultiply1/1 -> Sum of Elements/4
  Sum/1 -> Low-Pass Filter (Discrete or Continuous)/1
  e3/1 -> MatrixMultiply2/2
  V matrix/1(V) -> MATLAB Function1/1(V)
  MatrixMultiply4/1 -> Mux/1
  Mux/1 -> MatrixMultiply1/2, Gain1/1
  Current_Attitude/1 -> MATLAB Function4/1(states), H(q)/3(states), MATLAB Function/3(states)
  Current_Velocity/1 -> MatrixMultiply4/2
  MATLAB Function/1(G) -> Sum of Elements/2
  Selector1/1 -> Mux1/2
  Gain/1 -> MatrixMultiply/1
  inertia/1 -> H(q)/2(J), V matrix/1(J)
  Integrator/1 -> Sum of Elements/1, Sum/1
  Reciprocal/1 -> Gain/1
  H(q)/1(H) -> Sum1/1
  Sum of Elements/1 -> MatrixMultiply/2
  u/1 -> Selector1/1, Selector/1
  Gain1/1 -> Sum/2, Sum of Elements/5
  Sum1/1 -> Reciprocal/1
  Skew operator/1(S) -> V matrix/3(S)
  Product/1 -> MatrixMultiply2/1
  tilt/1 -> MATLAB Function2/1(tilt)
  H(q)/2(Q) -> Skew operator/1(Q), Derivative/1, V matrix/2(Q)
  MatrixMultiply2/1 -> Mux1/1
  gravity/1 -> MATLAB Function/2(g)
  Derivative/1 -> V matrix/4(Qdot)
  Transpose1/1 -> MatrixMultiply4/1
  Selector/1 -> Product/1
  MATLAB Function4/1(R) -> Transpose1/1
  mass/1 -> H(q)/1(m), MATLAB Function/1(m)
  Low-Pass Filter (Discrete or Continuous)/1 -> MATLAB Function3/1(u), est_force/1
  MATLAB Function3/1(y) -> dis_meas/1
